simulink model "aula3"  (R2018a)
settings: Solver=VariableStepAuto  StartTime=0.0  StopTime=10.0  RelTol=1e-3
values from neighbouring files (symbols this model uses):
  C = 1    [aula3.m]
  L = 1    [aula3.m]
  R = 1    [aula3.m]
settings Model: Creator=aluno  LastModifiedBy=aluno

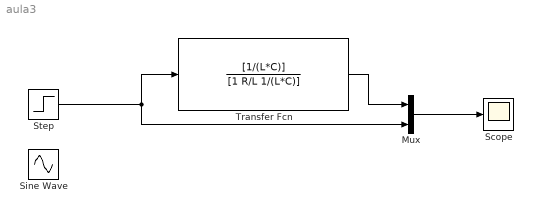
== system aula3 ==
  Mux : Mux  Inputs=2
  Scope : Scope
  Sine Wave : Sin  SampleTime=0
  Step : Step  SampleTime=0
  Transfer Fcn : TransferFcn  Numerator=[1/(L*C)]  Denominator=[1 R/L 1/(L*C)]
  wires:
  Step/1 -> Mux/2, Transfer Fcn/1
  Mux/1 -> Scope/1
  Transfer Fcn/1 -> Mux/1
